simulink model "PRBDM_3R_test001mdl"  (R2020b)
settings: Solver=ode113  StartTime=0.0  StopTime=T_f  RelTol=RT  AbsTol=AT  EnableMultiTasking=on
values from neighbouring files (symbols this model uses):
  kp = x(24)    [PRBDM_3R_CTC.m]    (also in PRBDM_3R_main.m = 20; PRBDM_3R_test001.m = 2; PRBDM_CTC_task.m = z(30); RRR_CTC.m)
  kv = x(23)    [PRBDM_3R_CTC.m]    (also in PRBDM_3R_main.m = 40; PRBDM_3R_test001.m = 4; PRBDM_CTC_task.m = z(29); RRR_CTC.m)
  L1 = z(8)    [Forward_kinematics.m]    (also in GeometricCalculation_simulink.m = Geoparams(5); Jacobi.m = x(4); PRBDM_3R_CTC.m = x(19); PRBDM_3R_Dynamic_Matrices_NewtonEular.m = robot_params(4))
  L2 = z(9)    [Forward_kinematics.m]    (also in GeometricCalculation_simulink.m = Geoparams(6); Jacobi.m = x(5); PRBDM_3R_CTC.m = x(20); PRBDM_3R_Dynamic_Matrices_NewtonEular.m = robot_params(5))
  L3 = z(10)    [Forward_kinematics.m]    (also in GeometricCalculation_simulink.m = Geoparams(7); Jacobi.m = x(6); PRBDM_3R_CTC.m = x(21); PRBDM_3R_Dynamic_Matrices_NewtonEular.m = robot_params(6))
  m1 = x(16)    [PRBDM_3R_CTC.m]    (also in PRBDM_3R_Dynamic_Matrices_NewtonEular.m = robot_params(1); PRBDM_3R_parameters.m = 0.35; PRBDM_3R_parameters.mat = 0.35; PRBDM_3R_test001.m = 0.1)
  m2 = x(17)    [PRBDM_3R_CTC.m]    (also in PRBDM_3R_Dynamic_Matrices_NewtonEular.m = robot_params(2); PRBDM_3R_parameters.m = 0.4; PRBDM_3R_parameters.mat = 0.4; PRBDM_3R_test001.m = 0.1)
  m3 = x(18)    [PRBDM_3R_CTC.m]    (also in PRBDM_3R_Dynamic_Matrices_NewtonEular.m = robot_params(3); PRBDM_3R_parameters.m = 0.15; PRBDM_3R_parameters.mat = 0.15; PRBDM_3R_test001.m = 0.1)
  W = x(22)    [PRBDM_3R_CTC.m]    (also in PRBDM_3R_Dynamic_Matrices_NewtonEular.m = robot_params(7); PRBDM_3R_Dynamics.m = in4dyn(20); PRBDM_3R_Dynamics00.m = in4dyn(20); PRBDM_3R_DynamicsPID.m = in4dyn(20))
settings Model: Creator=sayar  LastModifiedBy=Master
settings SolverCC: AutoScaleAbsTol=off
settings DataIOCC: SaveFormat=Array  ReturnWorkspaceOutputs=off  Refine=RF
settings OptimizationCC: ExpressionDepthLimit=2147483647  LifeSpan=inf
settings DebuggingCC: UnderspecifiedInitializationDetection=Classic  MergeDetectMultiDrivingBlocksExec=none  SolverPrmCheckMsg=warning  FcnCallInpInsideContextMsg=warning  StateNameClashWarn=warning  SFUnexpectedBacktrackingDiag=warning  SFNoUnconditionalDefaultTransitionDiag=warning  SFExecutionAtInitializationDiag=none  ArithmeticOperatorsInVariantConditions=warning
settings HardwareCC: ProdBitPerPointer=32  ProdBitPerSizeT=32  ProdBitPerPtrDiffT=32  ProdLargestAtomicFloat=None  ProdIntDivRoundTo=Undefined  ProdEndianess=Unspecified  ProdWordSize=32  ProdHWDeviceType=32-bit Generic
settings ModelReferenceCC: PropagateSignalLabelsOutOfModel=off
settings SFSimCC: SimUseLocalCustomCode=off  CustomCodeUndefinedFunction=UseInterfaceOnly
settings RTWCC: RTWUseLocalCustomCode=off
settings CodeAppCC: StateflowObjectComments=on
settings GRTTargetCC: TargetLangStandard=C89/C90 (ANSI)  CombineOutputUpdateFcns=off  GRTInterface=on
settings ConfigComp: CovMetricSettings=dw  CovSaveCumulativeToWorkspaceVar=on  CovSaveSingleToWorkspaceVar=on  CovExternalEMLEnable=off

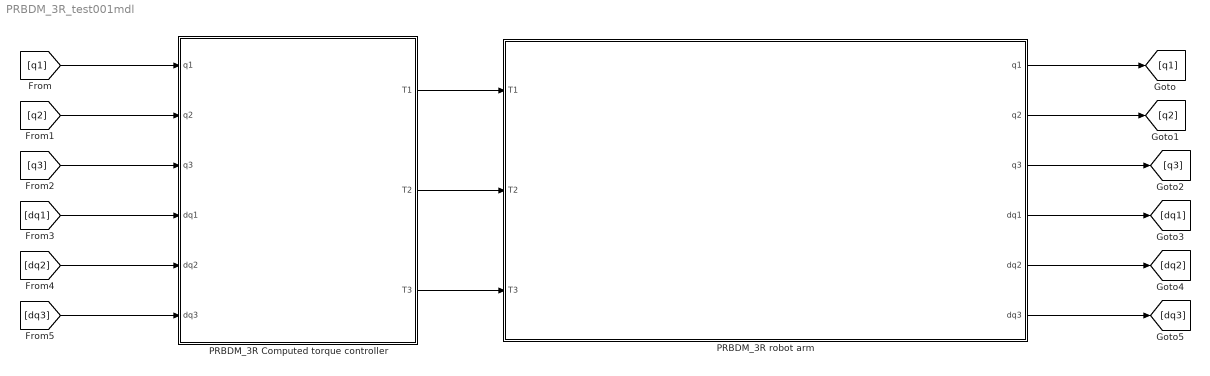
== system PRBDM_3R_test001mdl ==
  PRBDM_3R Computed torque controller : Subsystem
  PRBDM_3R robot arm : Subsystem
      mask Display: image(imread('RRR.png'))
  wires:
  [q1] -> PRBDM_3R Computed torque controller/1(q1)
  [q2] -> PRBDM_3R Computed torque controller/2(q2)
  [q3] -> PRBDM_3R Computed torque controller/3(q3)
  [dq1] -> PRBDM_3R Computed torque controller/4(dq1)
  [dq2] -> PRBDM_3R Computed torque controller/5(dq2)
  [dq3] -> PRBDM_3R Computed torque controller/6(dq3)
  PRBDM_3R Computed torque controller/1(T1) -> PRBDM_3R robot arm/1(T1)
  PRBDM_3R Computed torque controller/2(T2) -> PRBDM_3R robot arm/2(T2)
  PRBDM_3R Computed torque controller/3(T3) -> PRBDM_3R robot arm/3(T3)
  PRBDM_3R robot arm/1(q1) -> [q1]
  PRBDM_3R robot arm/2(q2) -> [q2]
  PRBDM_3R robot arm/3(q3) -> [q3]
  PRBDM_3R robot arm/4(dq1) -> [dq1]
  PRBDM_3R robot arm/5(dq2) -> [dq2]
  PRBDM_3R robot arm/6(dq3) -> [dq3]

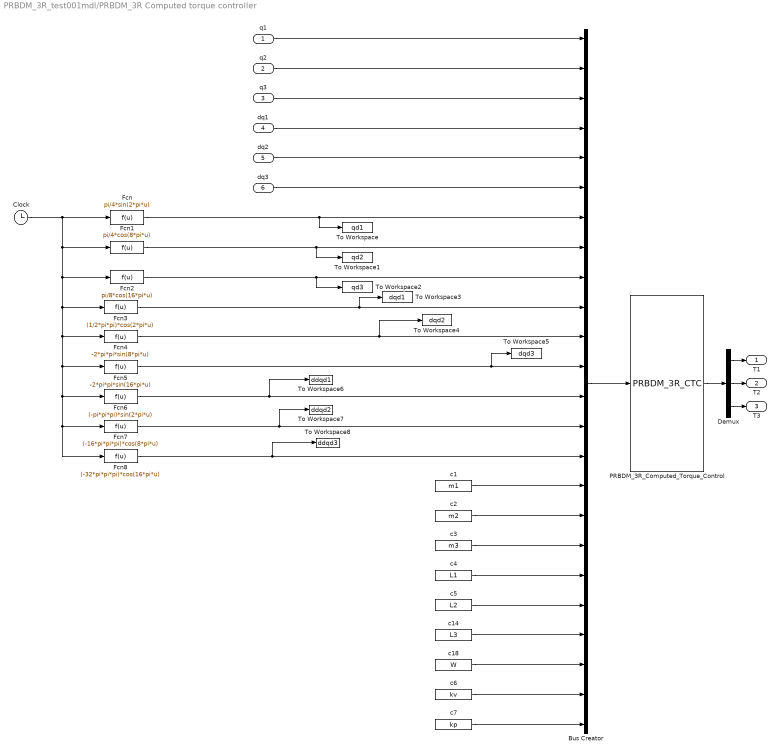
== system PRBDM_3R_test001mdl/PRBDM_3R Computed torque controller ==
  q1 : Inport
  q2 : Inport  Port=2
  q3 : Inport  Port=3
  dq1 : Inport  Port=4
  dq2 : Inport  Port=5
  dq3 : Inport  Port=6
  Bus Creator : BusCreator  Inputs=24
  Clock : Clock
  Demux : Demux  Outputs=3
  Fcn : Fcn  Expr=pi/4*sin(2*pi*u)
  Fcn1 : Fcn  Expr=pi/4*cos(8*pi*u)
  Fcn2 : Fcn  Expr=pi/8*cos(16*pi*u)
  Fcn3 : Fcn  Expr=(1/2*pi*pi)*cos(2*pi*u)
  Fcn4 : Fcn  Expr=-2*pi*pi*sin(8*pi*u)
  Fcn5 : Fcn  Expr=-2*pi*pi*sin(16*pi*u)
  Fcn6 : Fcn  Expr=(-pi*pi*pi)*sin(2*pi*u)
  Fcn7 : Fcn  Expr=(-16*pi*pi*pi)*cos(8*pi*u)
  Fcn8 : Fcn  Expr=(-32*pi*pi*pi)*cos(16*pi*u)
  PRBDM_3R_Computed_Torque_Control : MATLABFcn  MATLABFcn=PRBDM_3R_CTC  OutputDimensions=3
  To Workspace : ToWorkspace  VariableName=qd1  SampleTime=-1
  To Workspace1 : ToWorkspace  VariableName=qd2  SampleTime=-1
  To Workspace2 : ToWorkspace  VariableName=qd3  SampleTime=-1
  To Workspace3 : ToWorkspace  VariableName=dqd1  SampleTime=-1
  To Workspace4 : ToWorkspace  VariableName=dqd2  SampleTime=-1
  To Workspace5 : ToWorkspace  VariableName=dqd3  SampleTime=-1
  To Workspace6 : ToWorkspace  VariableName=ddqd1  SampleTime=-1
  To Workspace7 : ToWorkspace  VariableName=ddqd2  SampleTime=-1
  To Workspace8 : ToWorkspace  VariableName=ddqd3  SampleTime=-1
  c1 : Constant  Value=m1
  c14 : Constant  Value=L3
  c18 : Constant  Value=W
  c2 : Constant  Value=m2
  c3 : Constant  Value=m3
  c4 : Constant  Value=L1
  c5 : Constant  Value=L2
  c6 : Constant  Value=kv
  c7 : Constant  Value=kp
  T1 : Outport
  T2 : Outport  Port=2
  T3 : Outport  Port=3
  wires:
  PRBDM_3R_Computed_Torque_Control/1 -> Demux/1
  Bus Creator/1 -> PRBDM_3R_Computed_Torque_Control/1
  Demux/1 -> T1/1
  Demux/2 -> T2/1
  Demux/3 -> T3/1
  c1/1 -> Bus Creator/16
  c2/1 -> Bus Creator/17
  c3/1 -> Bus Creator/18
  c14/1 -> Bus Creator/21
  c18/1 -> Bus Creator/22
  q1/1 -> Bus Creator/1
  q2/1 -> Bus Creator/2
  q3/1 -> Bus Creator/3
  dq1/1 -> Bus Creator/4
  dq2/1 -> Bus Creator/5
  dq3/1 -> Bus Creator/6
  Clock/1 -> Fcn5/1, Fcn8/1, Fcn7/1, Fcn6/1, Fcn4/1, Fcn3/1, Fcn2/1, Fcn1/1, Fcn/1
  Fcn/1 -> To Workspace/1, Bus Creator/7
  Fcn1/1 -> Bus Creator/8, To Workspace1/1
  Fcn2/1 -> To Workspace2/1, Bus Creator/9
  Fcn3/1 -> To Workspace3/1, Bus Creator/10
  Fcn4/1 -> To Workspace4/1, Bus Creator/11
  Fcn5/1 -> To Workspace5/1, Bus Creator/12
  Fcn6/1 -> To Workspace6/1, Bus Creator/13
  Fcn7/1 -> To Workspace7/1, Bus Creator/14
  Fcn8/1 -> To Workspace8/1, Bus Creator/15
  c4/1 -> Bus Creator/19
  c5/1 -> Bus Creator/20
  c6/1 -> Bus Creator/23
  c7/1 -> Bus Creator/24

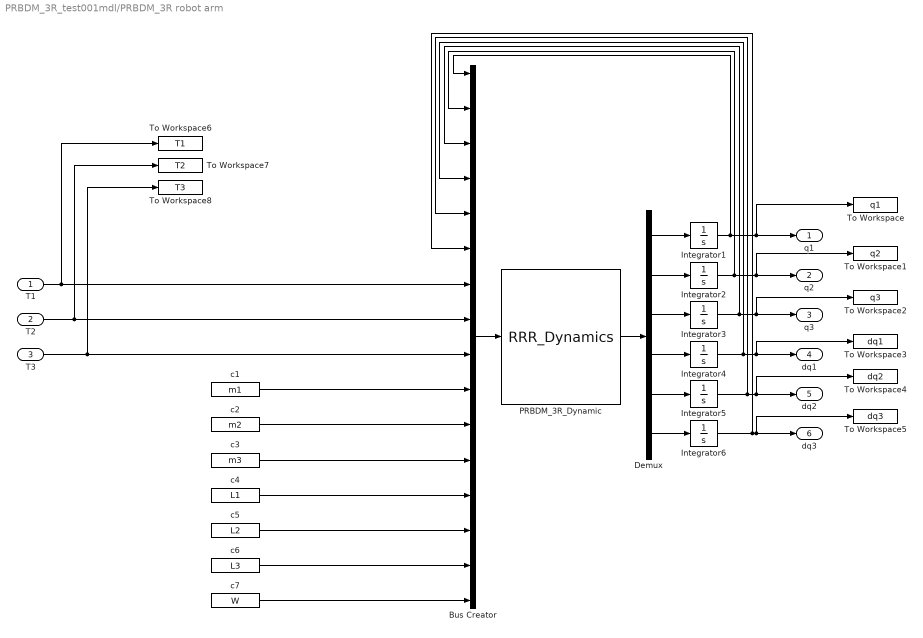
== system PRBDM_3R_test001mdl/PRBDM_3R robot arm ==
  T1 : Inport
  T2 : Inport  Port=2
  T3 : Inport  Port=3
  Bus Creator : BusCreator  Inputs=16
  Demux : Demux  Outputs=6
  Integrator{1,4..6} (4 alike) : Integrator
  Integrator2 : Integrator  InitialCondition=3*pi/4
  Integrator3 : Integrator  InitialCondition=-3*pi/4
  PRBDM_3R_Dynamic : MATLABFcn  MATLABFcn=RRR_Dynamics  OutputDimensions=6
  To Workspace : ToWorkspace  VariableName=q1  SampleTime=-1
  To Workspace1 : ToWorkspace  VariableName=q2  SampleTime=-1
  To Workspace2 : ToWorkspace  VariableName=q3  SampleTime=-1
  To Workspace3 : ToWorkspace  VariableName=dq1  SampleTime=-1
  To Workspace4 : ToWorkspace  VariableName=dq2  SampleTime=-1
  To Workspace5 : ToWorkspace  VariableName=dq3  SampleTime=-1
  To Workspace6 : ToWorkspace  VariableName=T1  SampleTime=-1
  To Workspace7 : ToWorkspace  VariableName=T2  SampleTime=-1
  To Workspace8 : ToWorkspace  VariableName=T3  SampleTime=-1
  c1 : Constant  Value=m1
  c2 : Constant  Value=m2
  c3 : Constant  Value=m3
  c4 : Constant  Value=L1
  c5 : Constant  Value=L2
  c6 : Constant  Value=L3
  c7 : Constant  Value=W
  q1 : Outport
  q2 : Outport  Port=2
  q3 : Outport  Port=3
  dq1 : Outport  Port=4
  dq2 : Outport  Port=5
  dq3 : Outport  Port=6
  wires:
  Demux/1 -> Integrator1/1
  Demux/2 -> Integrator2/1
  Demux/3 -> Integrator3/1
  Demux/4 -> Integrator4/1
  Demux/5 -> Integrator5/1
  Demux/6 -> Integrator6/1
  Integrator1/1 -> Bus Creator/1, q1/1, To Workspace/1
  Integrator2/1 -> Bus Creator/2, q2/1, To Workspace1/1
  Integrator3/1 -> Bus Creator/3, q3/1, To Workspace2/1
  Integrator4/1 -> Bus Creator/4, dq1/1, To Workspace3/1
  Integrator5/1 -> Bus Creator/5, dq2/1, To Workspace4/1
  Integrator6/1 -> Bus Creator/6, dq3/1, To Workspace5/1
  c1/1 -> Bus Creator/10
  c2/1 -> Bus Creator/11
  PRBDM_3R_Dynamic/1 -> Demux/1
  Bus Creator/1 -> PRBDM_3R_Dynamic/1
  T3/1 -> To Workspace8/1, Bus Creator/9
  T2/1 -> To Workspace7/1, Bus Creator/8
  T1/1 -> To Workspace6/1, Bus Creator/7
  c3/1 -> Bus Creator/12
  c4/1 -> Bus Creator/13
  c5/1 -> Bus Creator/14
  c6/1 -> Bus Creator/15
  c7/1 -> Bus Creator/16
